simulink model "SA_50"  (R2021a)
settings: Solver=VariableStepAuto  StartTime=0.0  StopTime=50  RelTol=1e-3
undefined symbols (not defined in the file or in its folder): Ion, Lithium, sigbuilder_block
libraries: spsCurrentMeasurementLib x3, spsSeriesRLCBranchLib x2, spsDiodeLib x2, spsBatteryLib x1, spsControlledCurrentSourceLib x1, spsFirstOrderFilterLib x1, spsFuelCellStackLib x1, spsMosfetLib x1, pid_lib x1, spsPWMGeneratorDCDCLib x1, spspowerguiLib x1
settings Model: SimulationMode=accelerator  Creator=g  LastModifiedBy=leonardopalacios
settings SolverCC: ZeroCrossAlgorithm=Adaptive  AlgebraicLoopSolver=TrustRegion
settings DataIOCC: ReturnWorkspaceOutputs=off
settings DebuggingCC: SFMachineParentedDataDiag=warning  ArithmeticOperatorsInVariantConditions=warning
settings SFSimCC: SimUseLocalCustomCode=off  CustomCodeUndefinedFunction=UseInterfaceOnly
settings RTWCC: RTWUseLocalCustomCode=off
settings CodeAppCC: StateflowObjectComments=on
settings SimscapeCC: SimscapeNormalizeSystem=off

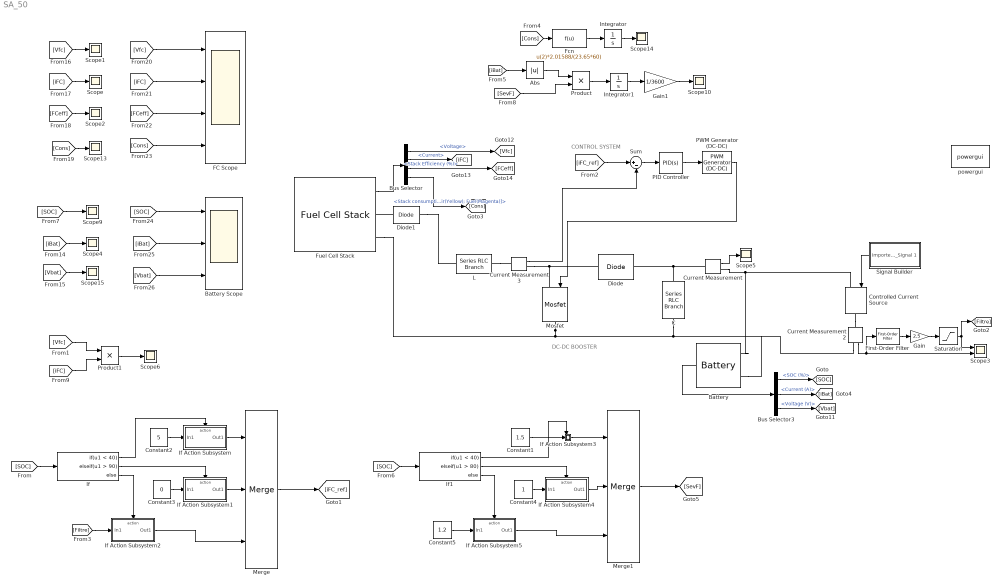
== system SA_50 ==
  note: CONTROL SYSTEM
  note: DC-DC BOOSTER
  Abs : Abs
  Battery : spsBatteryLib/Battery  BatType=Lithium-Ion  ShowTempParam=off  ThermalPreset=no  ShowAgeParam=off  NomV=40  NomQ=2.2  SOC=90  Batt_Tr=30  PresetModel=on  MaxQ=2.2  MinV=30  FullV=46.5595  Dis_rate=0.95652  R=0.18182  Normal_OP=1.9896  expZone="[43.2154     0.108087]"  current=[6.5 13 32.5]  Units=Time  Tci=20  NomT=25  T2=0  MaxQ2=2.208  FullV2=3.45  Normal_OP2=2.8  expZone2="[3.22        0.23]"  Rca=0.6  ti=1000  Dp=0  Neq0=0  Tsim=1e6  Ta1=25  Qeol=5.4*0.9  Reol=0.013333*1.2  Char_age=[2.3478, 3]  Dis_age=[2.3478, 10]  N1=1500  N2=10500  N3=1000  N4=1400  Ta2=45  N5=950
  "Battery Scope " : Scope  NumInputPorts=3
  Bus Selector : BusSelector  OutputSignals=Voltage,Current,Stack Efficiency (%),Stack consumption (Standard lpm) [Air(Yellow); Fuel(Magenta)]
  Bus Selector3 : BusSelector  OutputSignals=SOC (%),Current (A),Voltage (V)
  C : spsSeriesRLCBranchLib/Series RLC Branch  LConnTagsString=__new0  RConnTagsString=__new0  BranchType=C  Resistance=1  Inductance=100e-6  SetiL0=off  InitialCurrent=0  Capacitance=1000e-6  Setx0=off  InitialVoltage=0  Measurements=None
  Constant1 : Constant  Value=1.5
  Constant2 : Constant  Value=5
  Constant3 : Constant  Value=0
  Constant4 : Constant
  Constant5 : Constant  Value=1.2
  Controlled Current Source : spsControlledCurrentSourceLib/Controlled Current Source  Initialize=off  Source_Type=DC  Amplitude=0  Phase=0  Frequency=0  Measurements=Current
  Current Measurement : spsCurrentMeasurementLib/Current Measurement  PhasorSimulation=off  OutputType=Complex  PSBequivalent=0
  Current Measurement2 : spsCurrentMeasurementLib/Current Measurement  PhasorSimulation=off  OutputType=Complex  PSBequivalent=0
  Current Measurement3 : spsCurrentMeasurementLib/Current Measurement  PhasorSimulation=off  OutputType=Complex  PSBequivalent=0
  Diode : spsDiodeLib/Diode  Ron=0.001  Lon=0  Vf=0.8  IC=0  UseSnubber=off  Rs=500  Cs=250e-9  Measurements=off
  Diode1 : spsDiodeLib/Diode  Ron=0.001  Lon=0  Vf=0.8  IC=0  UseSnubber=off  Rs=500  Cs=250e-9  Measurements=off
  FC Scope : Scope  NumInputPorts=4
  Fcn : Fcn  Expr=u(2)*2.01588/(23.65*60)
  First-Order Filter : spsFirstOrderFilterLib/First-Order Filter  FilterType=Lowpass  Tc=5  Ts=0  Initialize=on  Vac_Init=[0, 0, 60]  Vdc_Init=1.1  PlotResponse=off  FreqRange="[0,  200,  1]"
  Fuel Cell Stack : spsFuelCellStackLib/Fuel Cell Stack  PresetModel=No (User-Defined)  FcType=0  Detailed=Detailed  Eoc="[18  15]"  NomVI="[4        12.5]"  EndVI="[5   12]"  Nc=20  n=46  TOp=25  AirFr=20  SuppPress="[0.35           0.3]"  Comp="[99.95           21            1]"  SignX=off  SignY=off  FlowRateH2=off  FlowRateAir=off  SystemTemp=off  SystemPH2=off  SystemPAir=off  FCDyn=off  FC_tau=1  Peak_O2=80  V_Under=10
      settings: SourceProductBaseCode=PS
  Gain : Gain  Gain=2.5
  Gain1 : Gain  Gain=1/3600
  If : If  IfExpression=u1 < 40  ElseIfExpressions=u1 > 90
  If Action Subsystem : Subsystem  TreatAsAtomicUnit=on
  If Action Subsystem1 : Subsystem  TreatAsAtomicUnit=on
  If Action Subsystem2 : Subsystem  TreatAsAtomicUnit=on
  If Action Subsystem3 : Subsystem  TreatAsAtomicUnit=on
  If Action Subsystem4 : Subsystem  TreatAsAtomicUnit=on
  If Action Subsystem5 : Subsystem  TreatAsAtomicUnit=on
  If1 : If  IfExpression=u1 < 40  ElseIfExpressions=u1 > 80
  Integrator : Integrator
  Integrator1 : Integrator
  L : spsSeriesRLCBranchLib/Series RLC Branch  LConnTagsString=__new0  RConnTagsString=__new0  BranchType=L  Resistance=1  Inductance=100e-3  SetiL0=off  InitialCurrent=0  Capacitance=1e-6  Setx0=off  InitialVoltage=0  Measurements=None
  Merge : Merge  Inputs=3
  Merge1 : Merge  Inputs=3
  Mosfet : spsMosfetLib/Mosfet  Ron=0.1  Lon=0  Rd=0.01  Vfd=0  IC=0  Rs=1e5  Cs=inf  Measurements=off
  PID Controller : pid_lib/PID Controller  Controller=PID  Form=Parallel  TimeDomain=Continuous-time  UseExternalTs=off  SampleTime=-1  IntegratorMethod=Forward Euler  FilterMethod=Forward Euler  ControllerParametersSource=internal  P=1  I=2  D=0  UseFilter=on  N=100  TunerSelectOption=Transfer Function Based (PID Tuner App)  InitialConditionSource=internal  InitialConditionForIntegrator=0  InitialConditionForFilter=0  DifferentiatorICPrevScaledInput=0  ExternalReset=none  TrackingMode=off  Kt=1  LimitOutput=off  SatLimitsSource=internal  UpperSaturationLimit=inf  LowerSaturationLimit=-inf  LinearizeAsGain=on  AntiWindupMode=none  Kb=1  POutMin=[]  POutMax=[]  IOutMin=[]  IOutMax=[]  DOutMin=[]  DOutMax=[]  NOutMin=[]  NOutMax=[]  SumOutMin=[]  SumOutMax=[]  SaturationOutMin=[]  SaturationOutMax=[]  PParamMin=[]  PParamMax=[]  IParamMin=[]  IParamMax=[]  DParamMin=[]  DParamMax=[]  NParamMin=[]  NParamMax=[]  KbParamMin=[]  KbParamMax=[]  KtParamMin=[]  KtParamMax=[]  KbOutMin=[]  KbOutMax=[]  KtOutMin=[]  KtOutMax=[]  IntegratorOutMin=[]  IntegratorOutMax=[]  FilterOutMin=[]  FilterOutMax=[]  SumI1OutMin=[]  SumI1OutMax=[]  SumI2OutMin=[]  SumI2OutMax=[]  SumI3OutMin=[]  SumI3OutMax=[]  SumI4OutMin=[]  SumI4OutMax=[]  SumDOutMin=[]  SumDOutMax=[]  DifferentiatorOutMin=[]  DifferentiatorOutMax=[]  FilterDiffOutCoefMin=[]  FilterDiffOutCoefMax=[]  ReciprocalOutMin=[]  ReciprocalOutMax=[]  SumDenOutMin=[]  SumDenOutMax=[]  SumNumOutMin=[]  SumNumOutMax=[]  DivideOutMin=[]  DivideOutMax=[]  UdiffTsProdOutMin=[]  UdiffTsProdOutMax=[]  NTsProdOutMin=[]  NTsProdOutMax=[]  UintegralTsProdOutMin=[]  UintegralTsProdOutMax=[]  UngainTsProdOutMin=[]  UngainTsProdOutMax=[]  IntegratorContinuousStateAttributes=''  IntegratorStateMustResolveToSignalObject=off  IntegratorRTWStateStorageClass=Auto  FilterContinuousStateAttributes=''  FilterStateMustResolveToSignalObject=off  FilterRTWStateStorageClass=Auto  ParallelPVariant=InternalParameters  IdealPVariant=Disabled  IVariant=InternalParameters  DVariant=InternalParameters  IntegratorVariant=Continuous  SatVariant=Disabled  AWVariant=Passthrough  PCopyVariant=Disabled  TRVariant=Disabled  FdbkBlocksVariant=Forward  IdealPFdbkVariant=Disabled  SatFdbkVariant=Disabled  DerivativeFilterVariant=ContFilter  NVariant=InternalParameters  NCopyVariant=Disabled  FilterICVariant=InternalICsFilter  IntegratorICVariant=InternalICs  ExternalResetVariant=Disabled  TRSumVariant=Passthrough  SumFdbkVariant=Disabled  SumVariant=Sum_PID  TsampFilterVariant=InternalTs  TsampNgainVariant=Passthrough  TsampIntegralVariant=Passthrough  ExternalSaturationOutDataTypeStr=Inherit: Same as second input
  PWM Generator (DC-DC) : spsPWMGeneratorDCDCLib/PWM Generator (DC-DC)  Fsw=1000  Ts=0
  Product : Product
  Product1 : Product
  Saturation : Saturate  UpperLimit=5  LowerLimit=0
  Scope{,1..2,4..6,9..10,13..15} (11 alike) : Scope
  Scope3 : Scope  NumInputPorts=2
  Signal Builder : Subsystem  Tag=STV Subsys  LoadFcn=sigbuilder_block('load');  StartFcn=sigbuilder_block('start');  StopFcn=sigbuilder_block('stop');  ClipboardFcn=sigbuilder_block('clipboard');  mask(Sigbuilder block){tuvar=[0:10]}
      mask help: Simulink:masks:SigbuilderBlock_MD
      mask init:
      | if ~strcmp(get_param(bdroot(gcbh),'SimulationStatus'),'stopped') tuvar = sigbuilder_block('maskInit'); end
      settings: CopyFcn=sigbuilder_block('copy');  DeleteFcn=sigbuilder_block('delete');  ModelCloseFcn=sigbuilder_block('modelClose');  PreSaveFcn=sigbuilder_block('preSave');  PauseFcn=sigbuilder_block('pause');  ContinueFcn=sigbuilder_block('continue');  NameChangeFcn=sigbuilder_block('namechange');  OpenFcn=sigbuilder_block('open',[298.2 169.8 514.8 208.8 ]);  CloseFcn=sigbuilder_block('close');
      mask Display: plot(0, 0, 100, 100,[2, 2, 32, 32, 2], [68, 8, 8, 68, 68],[32, 2], [38, 38], [32, 19, 2],[53, 60, 44], [32, 17, 17, 2],[16, 16, 31, 31]);txt = getActiveGroup(gcbh);text(2, 100, txt,'verticalAlignment', 'top');
  Sum : Sum  Inputs=|+-
  powergui : spspowerguiLib/powergui  Priority=1  SimulationMode=Continuous  SampleTime=50e-6  frequency=60  Iterations=50  frequencyindice=0  Pbase=100e6  ErrMax=1e-4  UnitsV=kV  UnitsW=MW  buscounter=0  FunctionMessages=off  echomessages=off  EnableUseOfTLC=off  CurrentSourceSwitches=off  DisableSnubberDevices=off  DisableRonSwitches=off  DisableVfSwitches=off  DisplayEquations=off  AutomaticDiscreteSolvers=off  SolverType=Tustin/Backward Euler (TBE)  Interpol=off  ExternalGateDelay=off  methode=off  Ts=10  x0status=blocks  SPID=off  SwTol=0  HookPort=off  NonlinearTolerance=1e-4  nMaxIteration=100  ContinueOnMaxIteration=off  RestoreLinks=warning  ResistiveCurrentMeasurement=off  Frange=[0:2:500]  Ylog=off  Xlog=on  ShowGrid=off  save=off  variable=ZData  structure=0  ZoomFFT=off  StartTime=0.0  cycles=1  DisplayStyle=1  fundamental=60  FreqAxis=off  MaxFrequency=1000  frequencyindicesteady=1  RmsSteady=1  display=off
  wires:
  Fuel Cell Stack/1 -> Bus Selector/1
  Current Measurement/1 -> Scope5/1
  Battery/1 -> Bus Selector3/1
  Current Measurement2/1 -> First-Order Filter/1, Scope3/2
  Signal Builder/1(Imported_Signal 1) -> Controlled Current Source/1
  [iFC_ref] -> Sum/1
  PWM Generator (DC-DC)/1 -> Mosfet/1
  Current Measurement3/1 -> Sum/2
  [SOC] -> If/1
  If/1 -> If Action Subsystem/Action
  If/2 -> If Action Subsystem1/Action
  If/3 -> If Action Subsystem2/Action
  Constant2/1 -> If Action Subsystem/1(In1)
  Constant3/1 -> If Action Subsystem1/1(In1)
  [Filtre] -> If Action Subsystem2/1(In1)
  If Action Subsystem/1(Out1) -> Merge/1
  If Action Subsystem1/1(Out1) -> Merge/2
  If Action Subsystem2/1(Out1) -> Merge/3
  Merge/1 -> [iFC_ref]
  First-Order Filter/1 -> Gain/1
  Saturation/1 -> [Filtre], Scope3/1
  [Cons] -> Fcn/1
  Fcn/1 -> Integrator/1
  Integrator/1 -> Scope14/1
  [iBat] -> Abs/1
  [SOC] -> If1/1
  If1/1 -> If Action Subsystem3/Action
  If1/2 -> If Action Subsystem4/Action
  If1/3 -> If Action Subsystem5/Action
  Constant1/1 -> If Action Subsystem3/1(In1)
  Constant4/1 -> If Action Subsystem4/1(In1)
  Constant5/1 -> If Action Subsystem5/1(In1)
  If Action Subsystem3/1(Out1) -> Merge1/1
  If Action Subsystem4/1(Out1) -> Merge1/2
  If Action Subsystem5/1(Out1) -> Merge1/3
  Merge1/1 -> [SevF]
  Abs/1 -> Product/1
  [SevF] -> Product/2
  Product/1 -> Integrator1/1
  Bus Selector/4 -> [Cons]  "<Stack consumption (Standard lpm) [Air(Yellow); Fuel(Magenta)]>"
  Bus Selector/1 -> [Vfc]  "<Voltage>"
  Bus Selector/2 -> [iFC]  "<Current>"
  Bus Selector/3 -> [FCeff]  "<Stack Efficiency (%)>"
  [SOC] -> Scope9/1
  [iBat] -> Scope4/1
  [Vbat] -> Scope15/1
  [Vfc] -> Scope1/1
  [iFC] -> Scope/1
  [FCeff] -> Scope2/1
  [Cons] -> Scope13/1
  [Vfc] -> FC Scope/1
  [iFC] -> FC Scope/2
  [FCeff] -> FC Scope/3
  [Cons] -> FC Scope/4
  [SOC] -> "Battery Scope "/1
  [iBat] -> "Battery Scope "/2
  [Vbat] -> "Battery Scope "/3
  Bus Selector3/1 -> [SOC]  "<SOC (%)>"
  Bus Selector3/2 -> [iBat]  "<Current (A)>"
  Bus Selector3/3 -> [Vbat]  "<Voltage (V)>"
  Sum/1 -> PID Controller/1
  PID Controller/1 -> PWM Generator (DC-DC)/1
  Gain/1 -> Saturation/1
  Integrator1/1 -> Gain1/1
  Gain1/1 -> Scope10/1
  [Vfc] -> Product1/1
  [iFC] -> Product1/2
  Product1/1 -> Scope6/1
  connections:
  Diode/LConn1 -- Current Measurement3/RConn1 -- Mosfet/LConn1
  C/LConn1 -- Current Measurement/LConn1 -- Diode/RConn1
  Mosfet/RConn1 -- Current Measurement2/RConn1 -- Battery/LConn2 -- C/RConn1 -- Fuel Cell Stack/RConn2
  Current Measurement/RConn1 -- Controlled Current Source/LConn1 -- Battery/LConn1
  Controlled Current Source/RConn1 -- Current Measurement2/LConn1
  L/RConn1 -- Current Measurement3/LConn1
  Diode1/LConn1 -- Fuel Cell Stack/RConn1
  Diode1/RConn1 -- L/LConn1

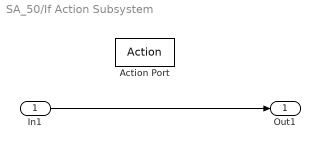
== system SA_50/If Action Subsystem ==
  In1 : Inport
  Action Port : ActionPort  ActionPortLabel=if(u1 < 40)
  Out1 : Outport
  wires:
  In1/1 -> Out1/1

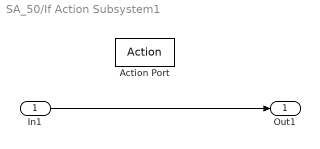
== system SA_50/If Action Subsystem1 ==
  In1 : Inport
  Action Port : ActionPort  ActionPortLabel=elseif(u1 > 90)
  Out1 : Outport
  wires:
  In1/1 -> Out1/1

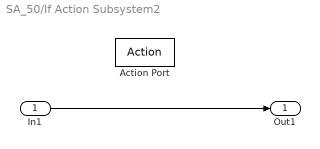
== system SA_50/If Action Subsystem2 ==
  In1 : Inport
  Action Port : ActionPort  ActionPortLabel=else
  Out1 : Outport
  wires:
  In1/1 -> Out1/1

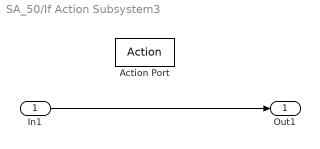
== system SA_50/If Action Subsystem3 ==
  In1 : Inport
  Action Port : ActionPort  ActionPortLabel=if(u1 < 40)
  Out1 : Outport
  wires:
  In1/1 -> Out1/1

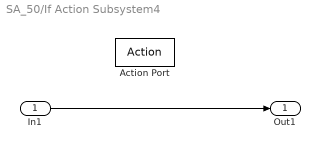
== system SA_50/If Action Subsystem4 ==
  In1 : Inport
  Action Port : ActionPort  ActionPortLabel=elseif(u1 > 80)
  Out1 : Outport
  wires:
  In1/1 -> Out1/1

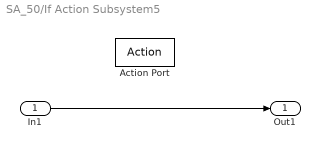
== system SA_50/If Action Subsystem5 ==
  In1 : Inport
  Action Port : ActionPort  ActionPortLabel=else
  Out1 : Outport
  wires:
  In1/1 -> Out1/1

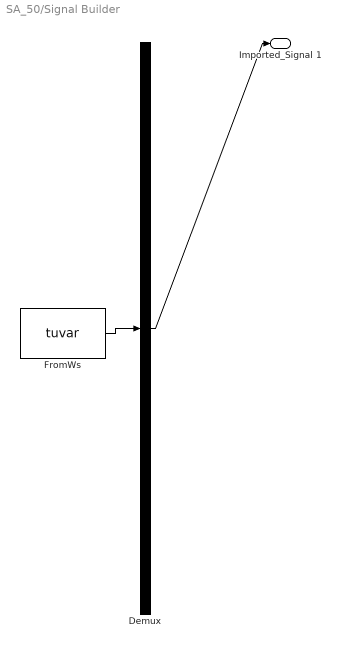
== system SA_50/Signal Builder ==
  Demux : Demux  Tag=STV Demux  Outputs=1
      settings: DisplayOption=none
  FromWs : FromWorkspace  Tag=STV FromWs  VariableName=tuvar
      SigBuilderData=|
      | common.afterFinalStr = 'Extrapolate'
      | common.sampleTime = 0
      | dataSet.timeRange = [0 1498.3]
      | dataSet.name = 'Combi12'
      | sbobj.Name = 'Signal Builder'
      | sbobj.Groups.Name = 'Combi12'
      | sbobj.Groups.Signals.Name = 'Imported_Signal 1'
      | sbobj.Groups.Signals.XData = [0 0.1 0.2 0.3 0.4 0.5 0.6 0.7 0.8 0.9 1 1.1 ... (14984 elements, 1x14984)]
      | sbobj.Groups.Signals.YData = [1.0569 1.1309 1.171 1.162 0.9589 1.143 1.056 1.261 1.1779 1.1458 1.2318 1.238 ... (14984 elements, 1x14984)]
      | sbobj.Groups.TimeRange = [0 1498.3]
  Imported_Signal 1 : Outport  Tag=STV Outport
  wires:
  FromWs/1 -> Demux/1
  Demux/1 -> Imported_Signal 1/1
